simulink model "SDRCapture"  (R2024b)
settings: Solver=VariableStepAuto  StartTime=0.0  StopTime=inf  FixedStep=0.1  RelTol=1e-3
libraries: commsdrhw_v2 x1
settings Model: Creator=lazar  LastModifiedBy=lazar
settings DataIOCC: ReturnWorkspaceOutputs=off

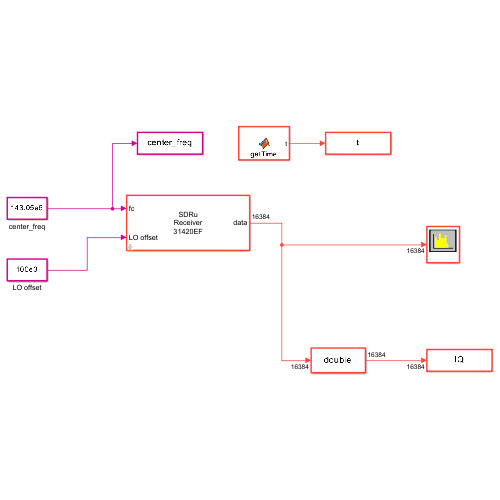
[thumbnail: Simulink's stored preview of the top-level diagram]
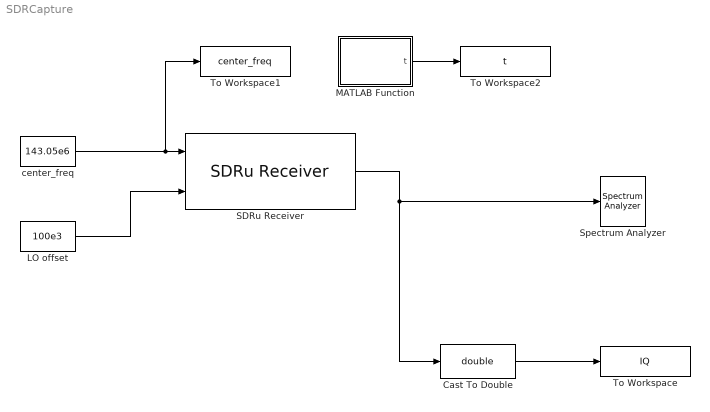
== system SDRCapture ==
  Cast To Double : DataTypeConversion  OutDataTypeStr=double  SaturateOnIntegerOverflow=off  RndMeth=Floor
  LO offset : Constant  Value=100e3
  MATLAB Function : MATLAB Function  TreatAsAtomicUnit=on
  SDRu Receiver : commsdrhw_v2/SDRu Receiver  rxtx=rx  initializeIPAddress=0  devMap=10  USRP2_IP=192.168.10.2  USRP_IP_X300=192.168.10.2  USRP_IP_X310=No devices found  USRP_IP_N300=192.168.10.2  USRP_IP_N310=192.168.10.2  USRP_IP_N320=192.168.10.2  USRP_serialNumB200=3136D21  USRP_serialNumB210=31420EF  platform=B210  prevPlatform=B210  lastIPAddressPopup=192.168.10.2  USRP_ID=31420EF  LastIPAddress=192.168.10.2  IsTwinRXDaughterboard=off  EnableTwinRXPhaseSync=off  losrc=0  ChannelMapping=1  centerFrequencySrc=Input port  centerFrequency=91.3e6  loOffsetSrc=Input port  loOffset=0  gainSrc=Dialog  gain=32  PPSSource=Internal  clockSource=Internal  EnableGPSLock=off  EnsureSyncGPSTime=off  EnableTimeTrigger=off  triggerTime=5  enableMIMOCableSync=off  EnableRefLock=off  masterClkRateParam=5000000  masterClkRateB200=32e6  masterClkRateB210=5e6  masterClkRateX300=200e6  masterClkRateX310=200e6  masterClkRateN300=125e6  masterClkRateN310=125e6  masterClkRateN320=200e6  masterClkRate=100e6  masterClkRateTwinRX=200e6  decimInterpSrc=Dialog  decimInterpPort=512  lastDecimSource=Dialog  decimInterp=80  USRP2_IP_NUM=[51 49 52 50 48 69 70]  sampleRate=62500  sampleTime=(80)/5000000  TransportDataType=int16  overrunUnderrunPort=off  dataLengthPort=off  EnableTimeStamps=off  outputDatatype=Same as transport data type  frameLength=2^14  HOST_DATA_PORT=0  HOST_CONTROL_PORT=0  USRP2_DATA_PORT=0  USRP2_CONTROL_PORT=0  bufferMode=Continuous streaming  EnableBurstMode=off  NumFramesInBurst=100
  Spectrum Analyzer : SpectrumAnalyzer  WindowPosition=[1.000000,49.000000,1680.000000,979.000000,]  Visible=on  ScopeFrameLocation=window  AxesScaling=Manual  FrequencyResolutionMethod=Number of frequency bands  WindowInvariantSamplesPerUpdate=on  FFTLength=2^15  Span=2500000  StartFrequency=-1250000  StopFrequency=1250000  ReferenceLoad=50  TimeResolution=0.3  TimeSpanSource=Property  TimeSpan=20  YLimits=[-26.36391639,8.01389685]  ColorLimits=[-12,-6]
  To Workspace : ToWorkspace  VariableName=IQ  SampleTime=-1
      settings: Save2DSignal=2-D array (concatenate along first dimension)
  To Workspace1 : ToWorkspace  VariableName=center_freq  SampleTime=-1
      settings: MaxDataPoints=1  Save2DSignal=2-D array (concatenate along first dimension)
  To Workspace2 : ToWorkspace  VariableName=t  SampleTime=-1
      settings: Save2DSignal=2-D array (concatenate along first dimension)
  center_freq : Constant  Value=143.05e6
  wires:
  center_freq/1 -> To Workspace1/1, SDRu Receiver/1
  LO offset/1 -> SDRu Receiver/2
  SDRu Receiver/1 -> Spectrum Analyzer/1, Cast To Double/1
  Cast To Double/1 -> To Workspace/1
  MATLAB Function/1(t) -> To Workspace2/1

== matlab function SDRCapture/MATLAB Function ==
  data: t output
function t = getTime()
% Returns current UTC time in seconds since UNIX epoch
% t = datetime('now','TimeZone','Local');
t = posixtime(datetime('now'));
end
